simulink model "Demo"  (Simulink 6.5)
settings: Solver=ode45  StartTime=0.0  StopTime=10.0  RelTol=1e-3
settings Model: Creator=suarezjl  LastModifiedBy=suarezjl
settings DataIOCC: SignalLoggingName=sigsOut
settings DebuggingCC: SolverPrmCheckMsg=none  MultiTaskDSMMsg=warning  MultiTaskCondExecSysMsg=none  StrictBusMsg=None
settings HardwareCC: TargetUnknown=on
settings RTWCC: IncludeERTFirstTime=on

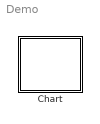
== system Demo ==
  Chart : Stateflow chart

== stateflow chart Chart ==
  state Start Cameras State Machine in Sally
    \\Sally\LeftReachDemo\HeadModule\LeftCameraAgent\StateMachine.LoadSM()
    \\Sally\LeftReachDemo\HeadModule\LeftCameraAgent\StateMachine.Start()
    \\Sally\LeftReachDemo\HeadModule\RightCameraAgent\StateMachine.LoadSM()
    \\Sally\LeftReachDemo\HeadModule\RightCameraAgent\StateMachine.Start()
    \\Sally\LeftReachDemo\HeadModule\RightCameraAgent\StateMachine.Wait(50)
  state Start Head
    \\Sally\LeftReachDemo\HeadModule\HeadAgent\StateMachine.LoadSM()
    \\Sally\LeftReachDemo\HeadModule\HeadAgent\StateMachine.Start()
    \\Sally\LeftReachDemo\HeadModule\HeadAgent\StateMachine.Wait(50)
  state Stop
    \\HungerForce\LeftReachDemo\LeftArm\StateMachine.Stop()
    \\HungerForce\LeftReachDemo\LeftTrajectoryAgent\StateMachine.Stop()
    \\HungerForce\LeftReachDemo\LeftArm\SampleIndPressure.Reset()
    \\Sally\LeftReachDemo\HeadModule\HeadAgent\StateMachine.Stop()
    \\Sally\LeftReachDemo\HeadModule\LeftCameraAgent\StateMachine.Stop()
    \\Sally\LeftReachDemo\HeadModule\RightCameraAgent\StateMachine.Stop()
  state Start Arm
    \\HungerForce\LeftReachDemo\LeftArm\StateMachine.LoadSM()
    \\HungerForce\LeftReachDemo\LeftArm\StateMachine.Start()
    \\HungerForce\LeftReachDemo\LeftArm\StateMachine.Wait(1000)
  Start Head -> Stop : Signal = "Stop"
  Start Cameras State Machine in Sally -> Start Head : Always
  (default) -> Start Arm : Start
  Start Arm -> Start Cameras State Machine in Sally : Always
